simulink model "altas"  (R2014a)
settings: Solver=ode45  StartTime=0.0  StopTime=10.0  RelTol=1e-3
libraries: fuzblock x1
settings Model: Creator=krish  LastModifiedBy=krish

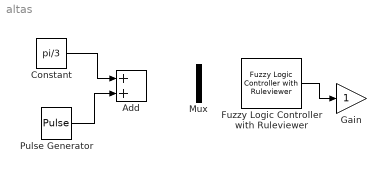
== system altas ==
  Add : Sum
  Constant : Constant  Value=pi/3
  Fuzzy Logic Controller with Ruleviewer : fuzblock/Fuzzy Logic  Controller  with Ruleviewer  fismatrix=[]  Ts=2
  Gain : Gain
  Mux : Mux  Inputs=2
  Pulse Generator : DiscretePulseGenerator  PulseType=Time based  Period=10  PulseWidth=5
  wires:
  Constant/1 -> Add/1
  Pulse Generator/1 -> Add/2
  Fuzzy Logic Controller with Ruleviewer/1 -> Gain/1
